simulink model "EnabledSubsystem_modelB"  (R2018b)
settings: Solver=FixedStepAuto  StartTime=0.0  StopTime=tFinal  FixedStep=deltaT  RelTol=1e-3
libraries: simulink x1
settings Model: Creator=Christopher  LastModifiedBy=Christopher

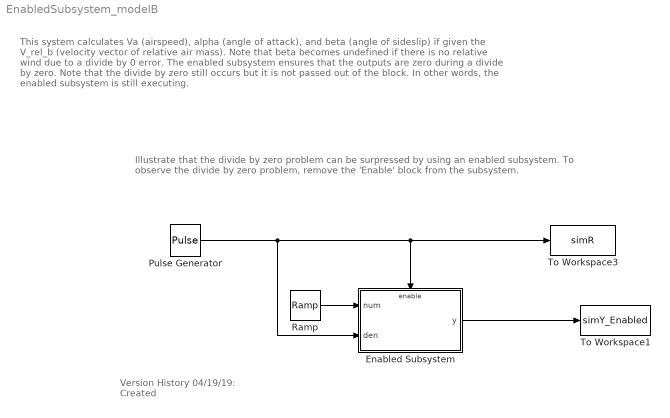
== system EnabledSubsystem_modelB ==
  note: Illustrate that the divide by zero problem can be surpressed by using an enabled subsystem.
      |
      | To observe the divide by zero problem, remove the 'Enable' block from the subsystem.
  note: This system calculates Va (airspeed), alpha (angle of attack), and beta (angle of sideslip) if given the V_rel_b (velocity vector of relative air mass).
      |
      | Note that beta becomes undefined if there is no relative wind due to a divide by 0 error.
      |
      | The enabled subsystem ensures that the outputs are zero during a divide by zero.  Note that the divide by zero still occurs but it is not passed out of the block.  In other words, the enabled subsystem is still executing.
  note: Version History
      | 04/19/19: Created
  Enabled Subsystem : Subsystem
  Pulse Generator : DiscretePulseGenerator  PulseType=Time based  Period=.5  PulseWidth=70
  Ramp : simulink/Sources/Ramp  slope=1  start=0  InitialOutput=0
  To Workspace1 : ToWorkspace  VariableName=simY_Enabled  SaveFormat=Timeseries  SampleTime=-1
  To Workspace3 : ToWorkspace  VariableName=simR  SaveFormat=Timeseries  SampleTime=-1
  wires:
  Pulse Generator/1 -> Enabled Subsystem/2(den), Enabled Subsystem/Enable, To Workspace3/1
  Enabled Subsystem/1(y) -> To Workspace1/1
  Ramp/1 -> Enabled Subsystem/1(num)

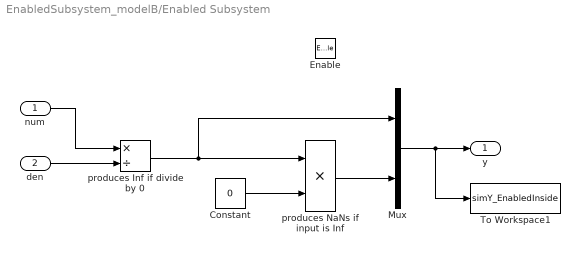
== system EnabledSubsystem_modelB/Enabled Subsystem ==
  num : Inport
  den : Inport  Port=2
  Enable : EnablePort
  Constant : Constant  Value=0
  Mux : Mux  Inputs=2
  To Workspace1 : ToWorkspace  VariableName=simY_EnabledInside  SaveFormat=Timeseries  SampleTime=-1
  produces Inf if divide by 0 : Product  Inputs=*/
  produces NaNs if input is Inf : Product
  y : Outport
  wires:
  den/1 -> produces Inf if divide by 0/2
  produces Inf if divide by 0/1 -> produces NaNs if input is Inf/1, Mux/1
  num/1 -> produces Inf if divide by 0/1
  produces NaNs if input is Inf/1 -> Mux/2
  Mux/1 -> y/1, To Workspace1/1
  Constant/1 -> produces NaNs if input is Inf/2
